simulink model "SimPrac9"  (R2018a)
settings: Solver=ode45  StartTime=0.0  StopTime=5  RelTol=1e-9
values from neighbouring files (symbols this model uses):
  K2 = 1/Kf    (= 24.2406840555)    [Prac9.m]
  Kg = Kfg*Kwg*Kag*Rng    [Prac9.m]
  Kr = 1/300    (= 0.00333333333333)    [Prac9.m]
  Ku = 50    [Prac9.m]
  Kusil = 1    [Prac9.m]
  T1 = J/(K1*Kf)    (= 0.00377725600536)    [Prac9.m]
  T1g = Tfg+ Tag    [Prac9.m]
  T2 = (Ta*T1)^0.5    (= 0.00378332483084)    [Prac9.m]
  T2g = (Tfg*Tag)^0.5    [Prac9.m]
  Ung = 110    [Prac9.m]
settings Model: Creator=dirlak  LastModifiedBy=dirlak

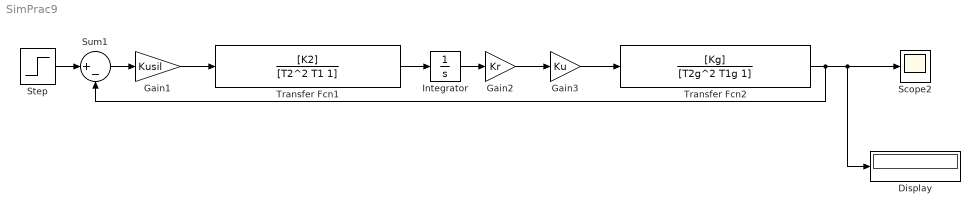
== system SimPrac9 ==
  Display : Display
  Gain1 : Gain  Gain=Kusil
  Gain2 : Gain  Gain=Kr
  Gain3 : Gain  Gain=Ku
  Integrator : Integrator
  Scope2 : Scope
  Step : Step  Time=0  After=Ung  SampleTime=0
  Sum1 : Sum  Inputs=|+-
  Transfer Fcn1 : TransferFcn  Numerator=[K2]  Denominator=[T2^2 T1 1]
  Transfer Fcn2 : TransferFcn  Numerator=[Kg]  Denominator=[T2g^2 T1g 1]
  wires:
  Step/1 -> Sum1/1
  Sum1/1 -> Gain1/1
  Gain1/1 -> Transfer Fcn1/1
  Gain2/1 -> Gain3/1
  Gain3/1 -> Transfer Fcn2/1
  Transfer Fcn2/1 -> Sum1/2, Display/1, Scope2/1
  Transfer Fcn1/1 -> Integrator/1
  Integrator/1 -> Gain2/1
